simulink model "uavopen_a"  (R2022b)
settings: Solver=VariableStepAuto  StartTime=0.0  StopTime=100  RelTol=1e-3
libraries: simulink x1
settings Model: Creator=Zzera  LastModifiedBy=Zzera

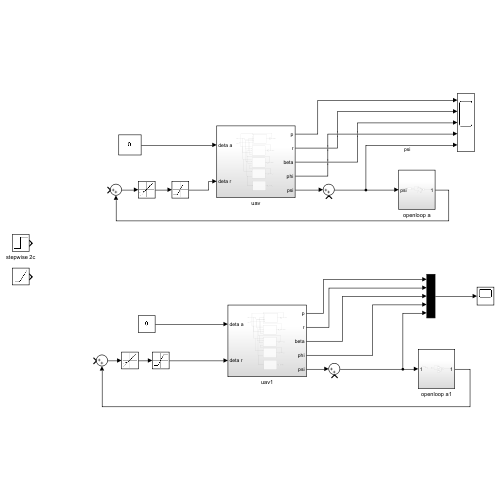
[thumbnail: Simulink's stored preview of the top-level diagram]
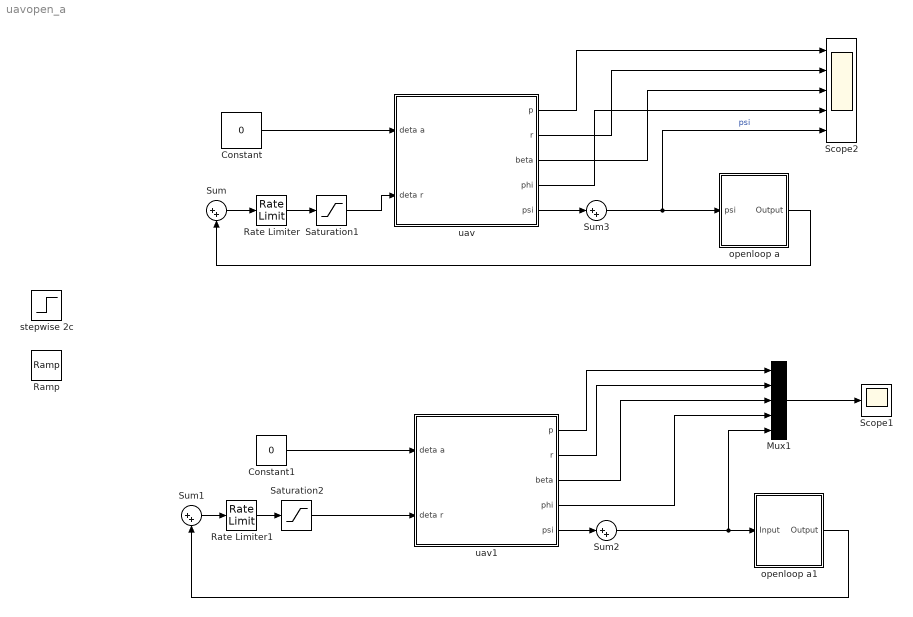
== system uavopen_a ==
  Constant : Constant  Value=0
  Constant1 : Constant  Value=0
  Mux1 : Mux  Inputs=5
  Ramp : simulink/Sources/Ramp  slope=0.1  start=0  InitialOutput=0
  Rate Limiter : RateLimiter  RisingSlewLimit=0.3491  FallingSlewLimit=-0.3491
  Rate Limiter1 : RateLimiter  RisingSlewLimit=0.3491  FallingSlewLimit=-0.3491
  Saturation1 : Saturate  UpperLimit=1.308  LowerLimit=-1.308
  Saturation2 : Saturate  UpperLimit=1.308  LowerLimit=-1.308
  Scope1 : Scope
  Scope2 : Scope  NumInputPorts=5
  Sum{,1..3} (4 alike) : Sum  Inputs=|++
  openloop a : Subsystem
  openloop a1 : Subsystem
  stepwise 2c : Step  After=0.2  SampleTime=10
  uav : Subsystem
  uav1 : Subsystem
  wires:
  Constant/1 -> uav/1(deta a)
  uav/2(r) -> Scope2/2
  uav/5(psi) -> Sum3/1
  uav/1(p) -> Scope2/1
  uav/3(beta) -> Scope2/3
  openloop a1/1(Output) -> Sum1/2
  uav1/3(beta) -> Mux1/3
  Constant1/1 -> uav1/1(deta a)
  uav1/5(psi) -> Sum2/1
  uav1/2(r) -> Mux1/2
  Mux1/1 -> Scope1/1
  uav1/4(phi) -> Mux1/4
  uav1/1(p) -> Mux1/1
  Sum2/1 -> Mux1/5, openloop a1/1(Input)
  Sum3/1 -> Scope2/5, openloop a/1(psi)  "psi"
  Saturation1/1 -> uav/2(deta r)
  Sum/1 -> Rate Limiter/1
  Rate Limiter/1 -> Saturation1/1
  Rate Limiter1/1 -> Saturation2/1
  Saturation2/1 -> uav1/2(deta r)
  Sum1/1 -> Rate Limiter1/1
  openloop a/1(Output) -> Sum/2
  uav/4(phi) -> Scope2/4

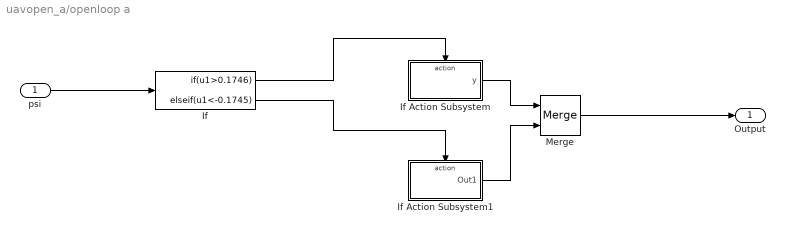
== system uavopen_a/openloop a ==
  psi : Inport
  If : If  IfExpression=u1>0.1746  ElseIfExpressions=u1<-0.1745  ShowElse=off
  If Action Subsystem : Subsystem  TreatAsAtomicUnit=on
  If Action Subsystem1 : Subsystem  TreatAsAtomicUnit=on
  Merge : Merge  InitialOutput=[0.3491]
  Output : Outport
  wires:
  psi/1 -> If/1
  If Action Subsystem/1(y) -> Merge/1
  If Action Subsystem1/1(Out1) -> Merge/2
  If/1 -> If Action Subsystem/Action
  If/2 -> If Action Subsystem1/Action
  Merge/1 -> Output/1

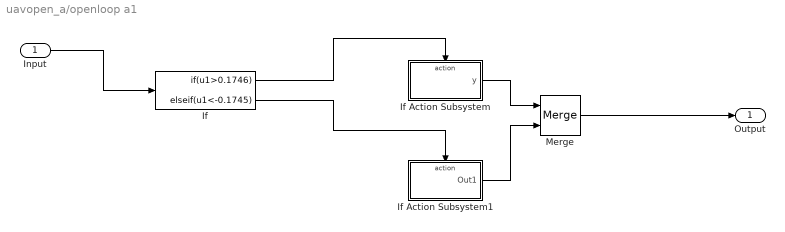
== system uavopen_a/openloop a1 ==
  Input : Inport
  If : If  IfExpression=u1>0.1746  ElseIfExpressions=u1<-0.1745  ShowElse=off
  If Action Subsystem : Subsystem  TreatAsAtomicUnit=on
  If Action Subsystem1 : Subsystem  TreatAsAtomicUnit=on
  Merge : Merge  InitialOutput=[0.3491]
  Output : Outport
  wires:
  Input/1 -> If/1
  If Action Subsystem/1(y) -> Merge/1
  If Action Subsystem1/1(Out1) -> Merge/2
  If/1 -> If Action Subsystem/Action
  If/2 -> If Action Subsystem1/Action
  Merge/1 -> Output/1

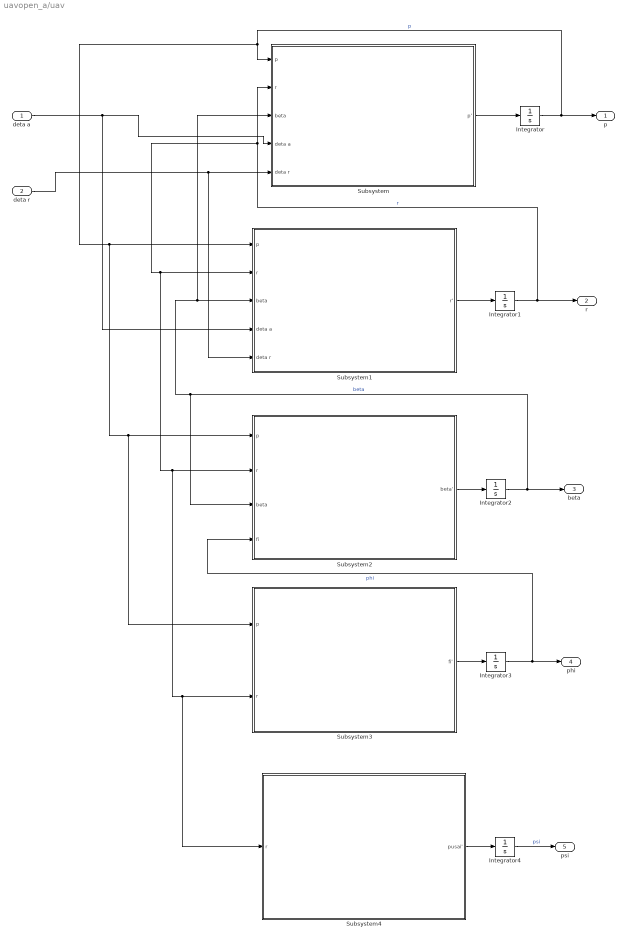
== system uavopen_a/uav ==
  deta a : Inport
  deta r : Inport  Port=2
  Integrator{,1..4} (5 alike) : Integrator
  Subsystem : Subsystem
  Subsystem1 : Subsystem
  Subsystem2 : Subsystem
  Subsystem3 : Subsystem
  Subsystem4 : Subsystem
  p : Outport
  r : Outport  Port=2
  beta : Outport  Port=3
  phi : Outport  Port=4
  psi : Outport  Port=5
  wires:
  Integrator4/1 -> psi/1  "psi"
  Integrator3/1 -> phi/1, Subsystem2/4(fi)  "phi"
  Subsystem/1(p') -> Integrator/1
  Subsystem3/1(fi') -> Integrator3/1
  Integrator/1 -> p/1, Subsystem3/1(p), Subsystem2/1(p), Subsystem1/1(p), Subsystem/1(p)  "p"
  Subsystem2/1(beta') -> Integrator2/1
  Integrator1/1 -> r/1, Subsystem/2(r), Subsystem4/1(r), Subsystem3/2(r), Subsystem2/2(r), Subsystem1/2(r)  "r"
  Subsystem4/1(pusai') -> Integrator4/1
  Integrator2/1 -> beta/1, Subsystem2/3(beta), Subsystem/3(beta), Subsystem1/3(beta)  "beta"
  Subsystem1/1(r') -> Integrator1/1
  deta a/1 -> Subsystem1/4(deta a), Subsystem/4(deta a)
  deta r/1 -> Subsystem1/5(deta r), Subsystem/5(deta r)

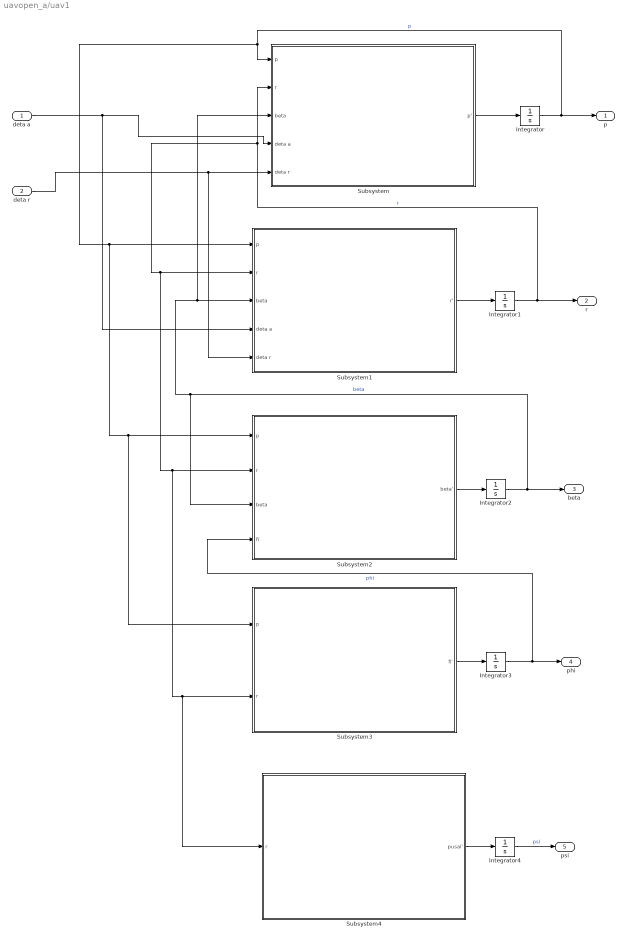
== system uavopen_a/uav1 ==
  deta a : Inport
  deta r : Inport  Port=2
  Integrator{,1..4} (5 alike) : Integrator
  Subsystem : Subsystem
  Subsystem1 : Subsystem
  Subsystem2 : Subsystem
  Subsystem3 : Subsystem
  Subsystem4 : Subsystem
  p : Outport
  r : Outport  Port=2
  beta : Outport  Port=3
  phi : Outport  Port=4
  psi : Outport  Port=5
  wires:
  Integrator4/1 -> psi/1  "psi"
  Integrator3/1 -> phi/1, Subsystem2/4(fi)  "phi"
  Subsystem/1(p') -> Integrator/1
  Subsystem3/1(fi') -> Integrator3/1
  Integrator/1 -> p/1, Subsystem3/1(p), Subsystem2/1(p), Subsystem1/1(p), Subsystem/1(p)  "p"
  Subsystem2/1(beta') -> Integrator2/1
  Integrator1/1 -> r/1, Subsystem/2(r), Subsystem4/1(r), Subsystem3/2(r), Subsystem2/2(r), Subsystem1/2(r)  "r"
  Subsystem4/1(pusai') -> Integrator4/1
  Integrator2/1 -> beta/1, Subsystem2/3(beta), Subsystem/3(beta), Subsystem1/3(beta)  "beta"
  Subsystem1/1(r') -> Integrator1/1
  deta a/1 -> Subsystem1/4(deta a), Subsystem/4(deta a)
  deta r/1 -> Subsystem1/5(deta r), Subsystem/5(deta r)

== system uavopen_a/openloop a/If Action Subsystem ==
  Action Port : ActionPort  ActionPortLabel=if(u1>0.1746)
  Constant : Constant  Value=-0.3491
  y : Outport
  wires:
  Constant/1 -> y/1

== system uavopen_a/openloop a/If Action Subsystem1 ==
  Action Port : ActionPort  ActionPortLabel=elseif(u1<-0.1745)
  Constant : Constant  Value=0.3491
  Out1 : Outport
  wires:
  Constant/1 -> Out1/1

== system uavopen_a/openloop a1/If Action Subsystem ==
  Action Port : ActionPort  ActionPortLabel=if(u1>0.1746)
  Constant : Constant  Value=-0.3491
  y : Outport
  wires:
  Constant/1 -> y/1

== system uavopen_a/openloop a1/If Action Subsystem1 ==
  Action Port : ActionPort  ActionPortLabel=elseif(u1<-0.1745)
  Constant : Constant  Value=0.3491
  Out1 : Outport
  wires:
  Constant/1 -> Out1/1

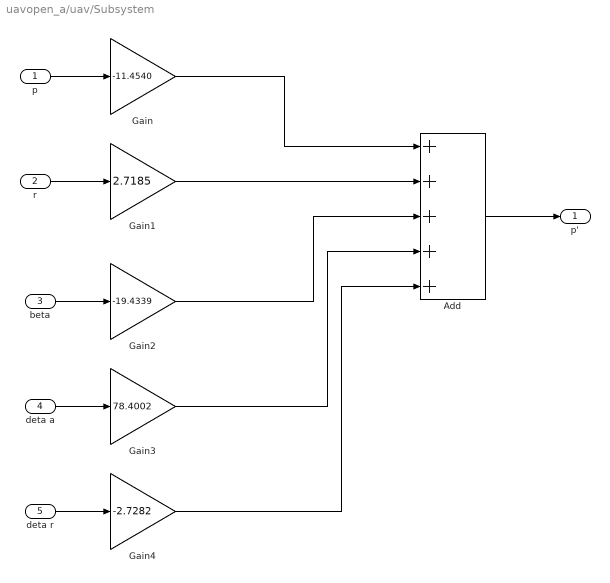
== system uavopen_a/uav/Subsystem ==
  p : Inport
  r : Inport  Port=2
  beta : Inport  Port=3
  deta a : Inport  Port=4
  deta r : Inport  Port=5
  Add : Sum  Inputs=+++++
  Gain : Gain  Gain=-11.4540
  Gain1 : Gain  Gain=2.7185
  Gain2 : Gain  Gain=-19.4339
  Gain3 : Gain  Gain=78.4002
  Gain4 : Gain  Gain=-2.7282
  p' : Outport
  wires:
  Gain2/1 -> Add/3
  Gain3/1 -> Add/4
  Gain/1 -> Add/1
  Gain1/1 -> Add/2
  Gain4/1 -> Add/5
  p/1 -> Gain/1
  r/1 -> Gain1/1
  beta/1 -> Gain2/1
  deta a/1 -> Gain3/1
  deta r/1 -> Gain4/1
  Add/1 -> p'/1

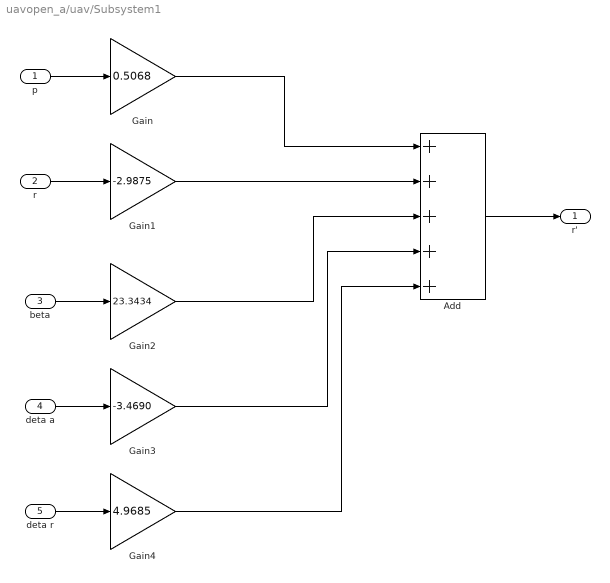
== system uavopen_a/uav/Subsystem1 ==
  p : Inport
  r : Inport  Port=2
  beta : Inport  Port=3
  deta a : Inport  Port=4
  deta r : Inport  Port=5
  Add : Sum  Inputs=+++++
  Gain : Gain  Gain=0.5068
  Gain1 : Gain  Gain=-2.9875
  Gain2 : Gain  Gain=23.3434
  Gain3 : Gain  Gain=-3.4690
  Gain4 : Gain  Gain=4.9685
  r' : Outport
  wires:
  p/1 -> Gain/1
  Gain4/1 -> Add/5
  Gain1/1 -> Add/2
  Gain/1 -> Add/1
  Gain2/1 -> Add/3
  beta/1 -> Gain2/1
  Gain3/1 -> Add/4
  deta a/1 -> Gain3/1
  Add/1 -> r'/1
  deta r/1 -> Gain4/1
  r/1 -> Gain1/1

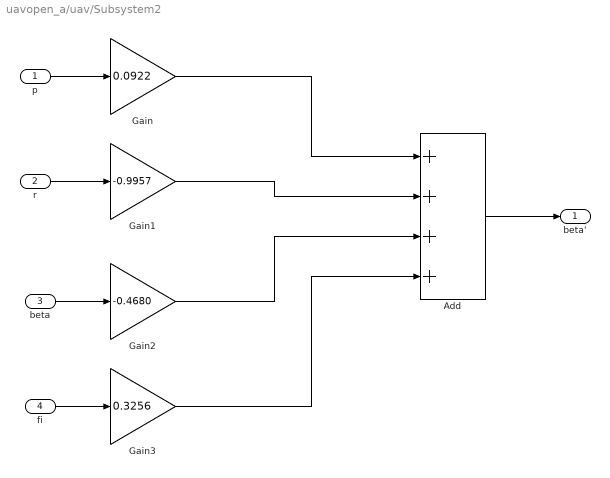
== system uavopen_a/uav/Subsystem2 ==
  p : Inport
  r : Inport  Port=2
  beta : Inport  Port=3
  fi : Inport  Port=4
  Add : Sum  Inputs=++++
  Gain : Gain  Gain=0.0922
  Gain1 : Gain  Gain=-0.9957
  Gain2 : Gain  Gain=-0.4680
  Gain3 : Gain  Gain=0.3256
  beta' : Outport
  wires:
  p/1 -> Gain/1
  Gain1/1 -> Add/2
  Gain/1 -> Add/1
  Gain2/1 -> Add/3
  beta/1 -> Gain2/1
  Gain3/1 -> Add/4
  fi/1 -> Gain3/1
  Add/1 -> beta'/1
  r/1 -> Gain1/1

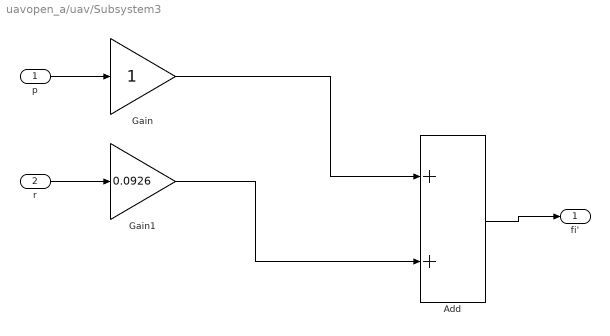
== system uavopen_a/uav/Subsystem3 ==
  p : Inport
  r : Inport  Port=2
  Add : Sum
  Gain : Gain
  Gain1 : Gain  Gain=0.0926
  fi' : Outport
  wires:
  p/1 -> Gain/1
  Gain1/1 -> Add/2
  Gain/1 -> Add/1
  Add/1 -> fi'/1
  r/1 -> Gain1/1

== system uavopen_a/uav/Subsystem4 ==
  r : Inport
  Gain1 : Gain
  pusai' : Outport
  wires:
  r/1 -> Gain1/1
  Gain1/1 -> pusai'/1

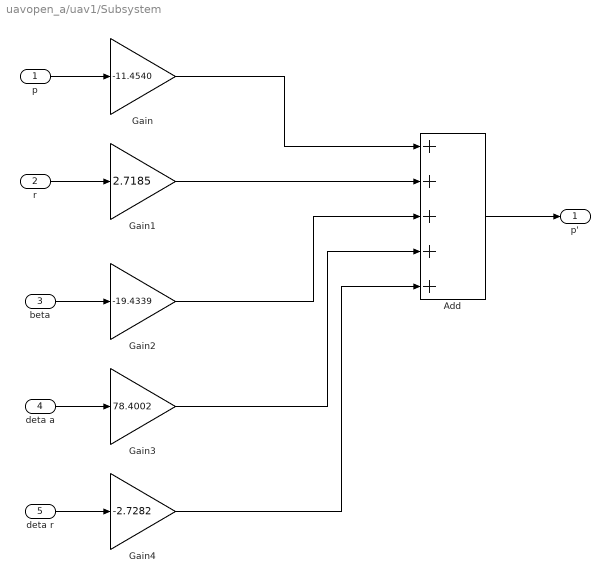
== system uavopen_a/uav1/Subsystem ==
  p : Inport
  r : Inport  Port=2
  beta : Inport  Port=3
  deta a : Inport  Port=4
  deta r : Inport  Port=5
  Add : Sum  Inputs=+++++
  Gain : Gain  Gain=-11.4540
  Gain1 : Gain  Gain=2.7185
  Gain2 : Gain  Gain=-19.4339
  Gain3 : Gain  Gain=78.4002
  Gain4 : Gain  Gain=-2.7282
  p' : Outport
  wires:
  Gain2/1 -> Add/3
  Gain3/1 -> Add/4
  Gain/1 -> Add/1
  Gain1/1 -> Add/2
  Gain4/1 -> Add/5
  p/1 -> Gain/1
  r/1 -> Gain1/1
  beta/1 -> Gain2/1
  deta a/1 -> Gain3/1
  deta r/1 -> Gain4/1
  Add/1 -> p'/1

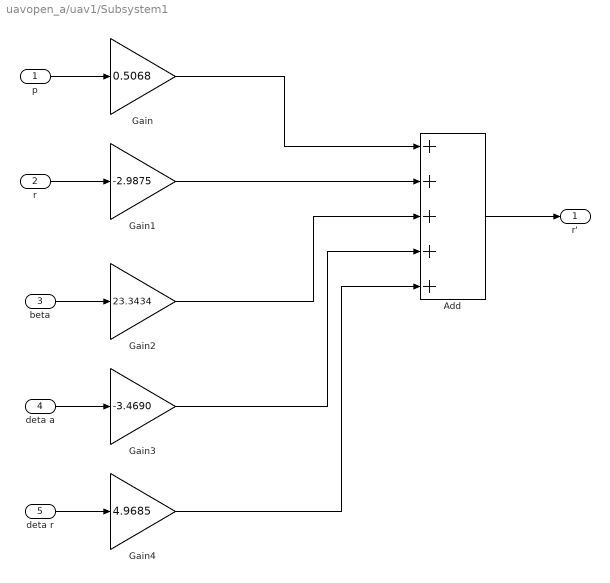
== system uavopen_a/uav1/Subsystem1 ==
  p : Inport
  r : Inport  Port=2
  beta : Inport  Port=3
  deta a : Inport  Port=4
  deta r : Inport  Port=5
  Add : Sum  Inputs=+++++
  Gain : Gain  Gain=0.5068
  Gain1 : Gain  Gain=-2.9875
  Gain2 : Gain  Gain=23.3434
  Gain3 : Gain  Gain=-3.4690
  Gain4 : Gain  Gain=4.9685
  r' : Outport
  wires:
  p/1 -> Gain/1
  Gain4/1 -> Add/5
  Gain1/1 -> Add/2
  Gain/1 -> Add/1
  Gain2/1 -> Add/3
  beta/1 -> Gain2/1
  Gain3/1 -> Add/4
  deta a/1 -> Gain3/1
  Add/1 -> r'/1
  deta r/1 -> Gain4/1
  r/1 -> Gain1/1

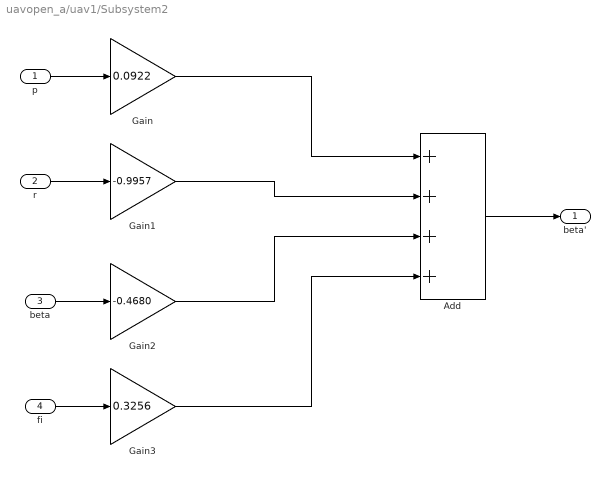
== system uavopen_a/uav1/Subsystem2 ==
  p : Inport
  r : Inport  Port=2
  beta : Inport  Port=3
  fi : Inport  Port=4
  Add : Sum  Inputs=++++
  Gain : Gain  Gain=0.0922
  Gain1 : Gain  Gain=-0.9957
  Gain2 : Gain  Gain=-0.4680
  Gain3 : Gain  Gain=0.3256
  beta' : Outport
  wires:
  p/1 -> Gain/1
  Gain1/1 -> Add/2
  Gain/1 -> Add/1
  Gain2/1 -> Add/3
  beta/1 -> Gain2/1
  Gain3/1 -> Add/4
  fi/1 -> Gain3/1
  Add/1 -> beta'/1
  r/1 -> Gain1/1

== system uavopen_a/uav1/Subsystem3 ==
  p : Inport
  r : Inport  Port=2
  Add : Sum
  Gain : Gain
  Gain1 : Gain  Gain=0.0926
  fi' : Outport
  wires:
  p/1 -> Gain/1
  Gain1/1 -> Add/2
  Gain/1 -> Add/1
  Add/1 -> fi'/1
  r/1 -> Gain1/1

== system uavopen_a/uav1/Subsystem4 ==
  r : Inport
  Gain1 : Gain
  pusai' : Outport
  wires:
  r/1 -> Gain1/1
  Gain1/1 -> pusai'/1
